simulink model "FORWARD_KINEMATICS_DUY"  (R2016a)
settings: Solver=VariableStepAuto  StartTime=0.0  StopTime=5  MaxStep=0.01  RelTol=1e-3
values from neighbouring files (symbols this model uses):
  phi = [phi1; phi2; phi3]    [Inverse_Dynamic_Model.m]    (also in Inverse_Dynamic_Model_Test_Result.m; Kinematic_Dimension.m; _PARAMETER_OF_DELTA_ROBOT.m)
  r = r1- r2    (= 150)    [FORWARD_KINEMATICS_DELTA_ROBOT.m]    (also in Inverse_Dynamic_Model.m = -0.15; Inverse_Dynamic_Model_Test_Result.m = -0.15; Kinematic_Dimension.m; _PARAMETER_OF_DELTA_ROBOT.m = -0.15)
undefined symbols (not defined in the file or in its folder): R
settings Model: Creator=computer  LastModifiedBy=ThanhUTC
settings DataIOCC: SaveFormat=Array

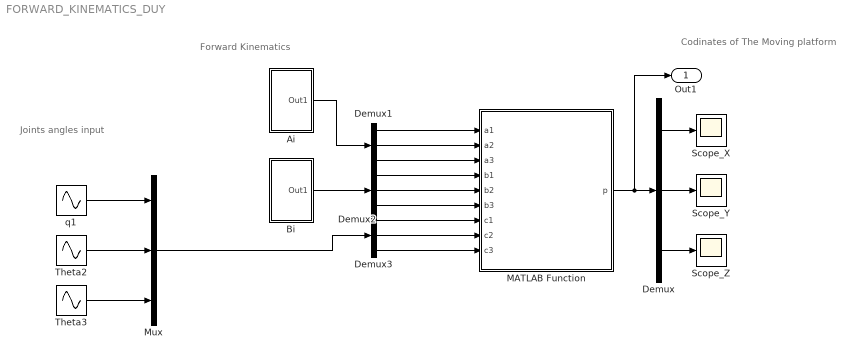
== system FORWARD_KINEMATICS_DUY ==
  note: Forward Kinematics
  note: Codinates of The Moving platform
  note: Joints angles input
  Ai : Subsystem
  Bi : Subsystem
  Demux{,1..3} (4 alike) : Demux  Outputs=3
  MATLAB Function : MATLAB Function  TreatAsAtomicUnit=on
  Mux : Mux  Inputs=3
  Scope_X : Scope
  Scope_Y : Scope
  Scope_Z : Scope
  Theta2 : Sin  Amplitude=0.5  Bias=pi/8  Frequency=pi/2  SampleTime=0
  Theta3 : Sin  Amplitude=0.5  Frequency=pi  SampleTime=0
  q1 : Sin  Frequency=1.5  SampleTime=0
  Out1 : Outport
  wires:
  Theta2/1 -> Mux/2
  q1/1 -> Mux/1
  Theta3/1 -> Mux/3
  Demux/3 -> Scope_Z/1
  Demux/2 -> Scope_Y/1
  Demux/1 -> Scope_X/1
  MATLAB Function/1(p) -> Out1/1, Demux/1
  Demux3/2 -> MATLAB Function/8(c2)
  Demux3/1 -> MATLAB Function/7(c1)
  Demux3/3 -> MATLAB Function/9(c3)
  Demux2/1 -> MATLAB Function/4(b1)
  Demux2/3 -> MATLAB Function/6(b3)
  Ai/1(Out1) -> Demux1/1
  Demux2/2 -> MATLAB Function/5(b2)
  Mux/1 -> Demux3/1
  Demux1/2 -> MATLAB Function/2(a2)
  Demux1/1 -> MATLAB Function/1(a1)
  Demux1/3 -> MATLAB Function/3(a3)
  Bi/1(Out1) -> Demux2/1

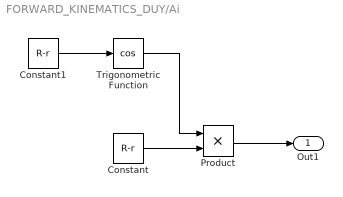
== system FORWARD_KINEMATICS_DUY/Ai ==
  Constant : Constant  Value=R-r
  Constant1 : Constant  Value=R-r
  Product : Product
  Trigonometric Function : Trigonometry  Operator=cos
  Out1 : Outport
  wires:
  Constant/1 -> Product/2
  Constant1/1 -> Trigonometric Function/1
  Trigonometric Function/1 -> Product/1
  Product/1 -> Out1/1

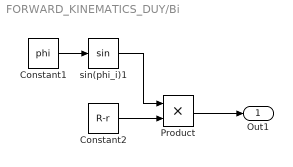
== system FORWARD_KINEMATICS_DUY/Bi ==
  Constant1 : Constant  Value=phi
  Constant2 : Constant  Value=R-r
  Product : Product
  sin(phi_i)1 : Trigonometry
  Out1 : Outport
  wires:
  Constant1/1 -> sin(phi_i)1/1
  Constant2/1 -> Product/2
  sin(phi_i)1/1 -> Product/1
  Product/1 -> Out1/1

== matlab function FORWARD_KINEMATICS_DUY/MATLAB Function ==
  data: p output; a1 input; a2 input; a3 input; b1 input; b2 input; b3 input; c1 input; c2 input; c3 input
function p = equasol(a1, a2, a3, b1, b2, b3, c1, c2, c3)
%#codegen
 coder.extrinsic('solequa'); 
 p = zeros(3,1);
 p = solequa(a1, a2, a3, b1, b2, b3, c1, c2, c3);
